simulink model "hw3_2c"  (R2022b)
settings: Solver=VariableStepAuto  StartTime=0.0  StopTime=60  RelTol=1e-3
undefined symbols (not defined in the file): b, k, m
settings Model: Creator=gaura  LastModifiedBy=gaura

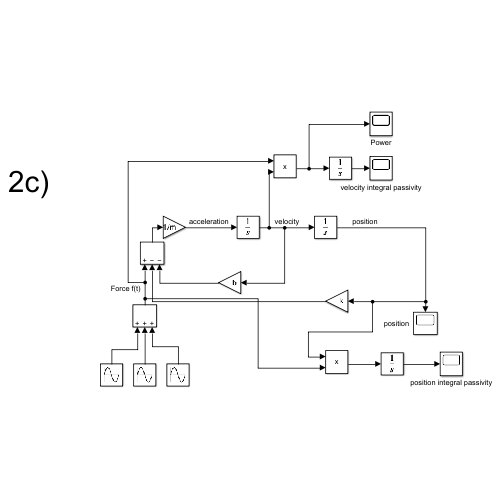
[thumbnail: Simulink's stored preview of the top-level diagram]
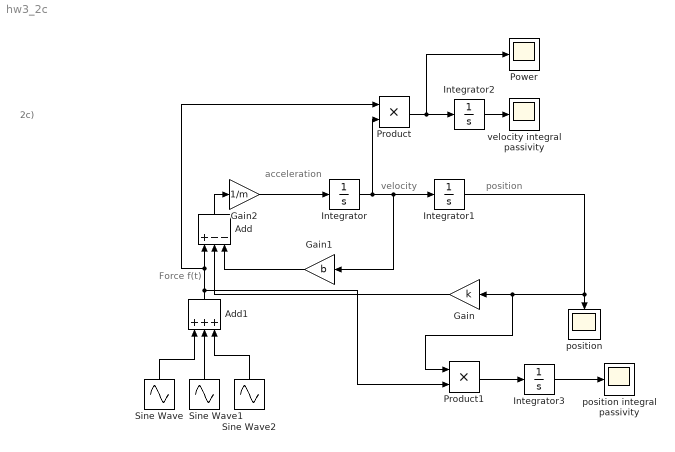
== system hw3_2c ==
  note: Force f(t)
  note: acceleration
  note: position
  note: velocity
  note: 2c)
  Add : Sum  Inputs=+--
  Add1 : Sum  Inputs=+++
  Gain : Gain  Gain=k
  Gain1 : Gain  Gain=b
  Gain2 : Gain  Gain=1/m
  Integrator{,1..3} (4 alike) : Integrator
  Power : Scope
  Product : Product
  Product1 : Product
  Sine Wave : Sin  Amplitude=20  SampleTime=0
  Sine Wave1 : Sin  Amplitude=10  Frequency=2  Phase=pi/2  SampleTime=0
  Sine Wave2 : Sin  Amplitude=20  Frequency=10  SampleTime=0
  position : Scope
  position integral passivity : Scope
  velocity integral passivity : Scope
  wires:
  Integrator/1 -> Product/2, Gain1/1, Integrator1/1
  Integrator1/1 -> Product1/1, Gain/1, position/1
  Gain/1 -> Add/2
  Gain1/1 -> Add/3
  Add/1 -> Gain2/1
  Add1/1 -> Product1/2, Product/1, Add/1
  Sine Wave2/1 -> Add1/3
  Sine Wave1/1 -> Add1/2
  Sine Wave/1 -> Add1/1
  Gain2/1 -> Integrator/1
  Product/1 -> Power/1, Integrator2/1
  Integrator2/1 -> velocity integral passivity/1
  Product1/1 -> Integrator3/1
  Integrator3/1 -> position integral passivity/1
